simulink model "model_sim"  (R2024b)
settings: Solver=FixedStepAuto  StartTime=0.0  StopTime=tsim  FixedStep=T  RelTol=1e-3
settings Model: Creator=usuario  LastModifiedBy=usuario
settings DataIOCC: ReturnWorkspaceOutputs=off  TimeSaveName=t
settings RTWCC: GPUComputeCapability=3.5

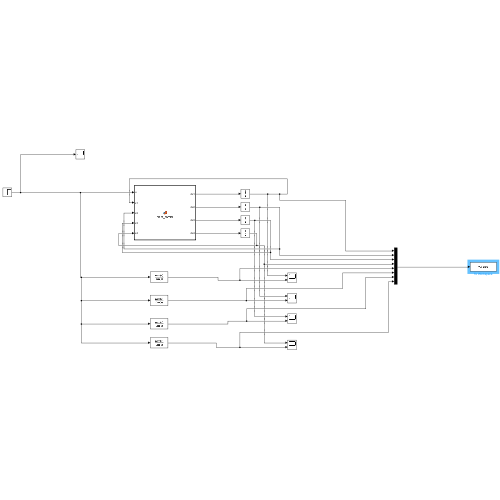
[thumbnail: Simulink's stored preview of the top-level diagram]
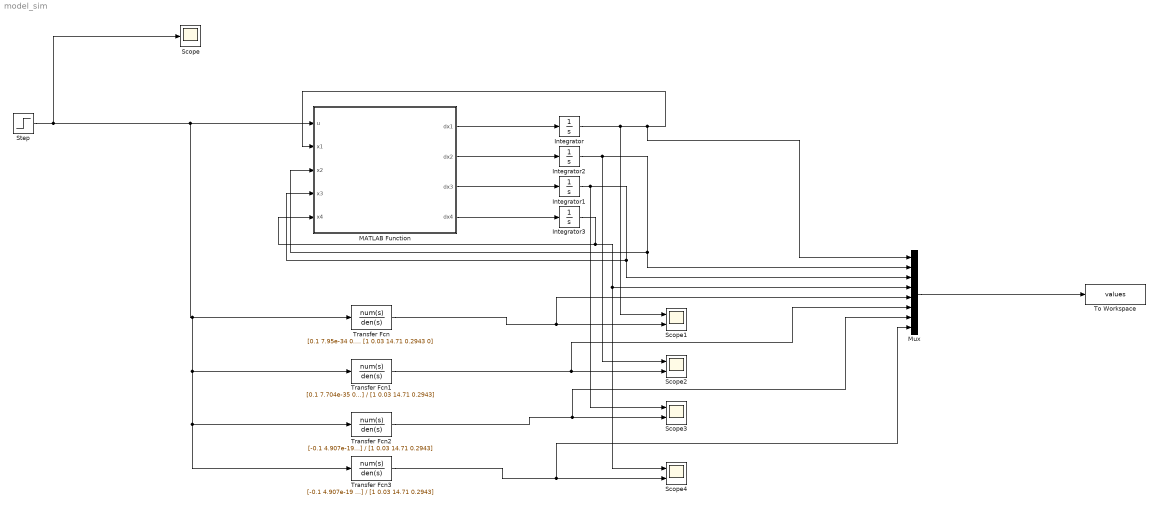
== system model_sim ==
  Integrator : Integrator  InitialCondition=0.002
  Integrator1 : Integrator  InitialCondition=0.001
  Integrator2 : Integrator
  Integrator3 : Integrator
  MATLAB Function : MATLAB Function  TreatAsAtomicUnit=on
  Mux : Mux  Inputs=8
  Scope : Scope
  Scope{1..4} (4 alike) : Scope  NumInputPorts=2
  Step : Step  After=5  SampleTime=0
  To Workspace : ToWorkspace  VariableName=values  SampleTime=-1
  Transfer Fcn : TransferFcn  Numerator=[0.1 7.95e-34 0.981]  Denominator=[1 0.03 14.71 0.2943 0]
  Transfer Fcn1 : TransferFcn  Numerator=[0.1 7.704e-35 0.981]  Denominator=[1 0.03 14.71 0.2943]
  Transfer Fcn2 : TransferFcn  Numerator=[-0.1 4.907e-19]  Denominator=[1 0.03 14.71 0.2943]
  Transfer Fcn3 : TransferFcn  Numerator=[-0.1 4.907e-19 3.057e-37]  Denominator=[1 0.03 14.71 0.2943]
  wires:
  Mux/1 -> To Workspace/1
  MATLAB Function/1(dx1) -> Integrator/1
  Integrator2/1 -> Scope2/1, Mux/2, MATLAB Function/3(x2)
  Integrator3/1 -> MATLAB Function/5(x4), Scope4/1, Mux/4
  Integrator/1 -> Scope1/1, Mux/1, MATLAB Function/2(x1)
  Integrator1/1 -> Scope3/1, MATLAB Function/4(x3), Mux/3
  MATLAB Function/3(dx3) -> Integrator1/1
  MATLAB Function/4(dx4) -> Integrator3/1
  MATLAB Function/2(dx2) -> Integrator2/1
  Step/1 -> Scope/1, Transfer Fcn3/1, Transfer Fcn2/1, Transfer Fcn1/1, Transfer Fcn/1, MATLAB Function/1(u)
  Transfer Fcn/1 -> Mux/5, Scope1/2
  Transfer Fcn1/1 -> Mux/6, Scope2/2
  Transfer Fcn2/1 -> Mux/7, Scope3/2
  Transfer Fcn3/1 -> Mux/8, Scope4/2

== matlab function model_sim/MATLAB Function ==
  data: u input; dx1 output; x1 input; x2 input; x3 input; x4 input; dx2 output; dx3 output; dx4 output
function [dx1,dx2,dx3,dx4] = plant_model(u,x1,x2,x3,x4)
M = 10;g=9.8;m=5;l=1;mu=0.3;
q = [x1;x2;x3;x4];
a11 = -mu/(M+m*sin(x3)^2); a12 = m*g*cos(x3)*sin(x3)/((M+m*sin(x3)^2)*x3);
a13 = m*l*x4*sin(x3)/(M+m*sin(x3)^2); a21 = mu*cos(x3)/(l*(M+m*sin(x3)^2));
a22 = -(M+m)*g*sin(x3)/(l*x3*(M+m*sin(x3)^2)); a23=-m*x4*sin(x3)*cos(x3)/(M+m*sin(x3)^2);
b1 = 1/(M+m*sin(x3)^2); b2 = -cos(x3)/(l*(M+m*sin(x3)^2));
A = [0 1 0 0;0 a11 a12 a13;0 0 0 1;0 a21 a22 a23];
B = [0;b1;0;b2];

dq = A*q + B*u;
dx1 = dq(1);
dx2 = dq(2);
dx3 = dq(3);
dx4 = dq(4);
